simulink model "openWaterModel"  (R2020a)
settings: Solver=FixedStepAuto  StartTime=0.0  StopTime=inf  FixedStep=Ts  RelTol=1e-3  EnableMultiTasking=on
values from neighbouring files (symbols this model uses):
  ctrlMap =     [init_Kite.mat]
  Ts = 0.01    [init_Kite.mat]
undefined symbols (not defined in the file or in its folder): initializeBussesFromBlock, IO397, standard
libraries: xpcutilitieslib x172, hdlsllib x100, simulink x36, dspsigops x13, slrtlib x4, xpcseriallib x3, speedgoatlib_fpga_analog_io x2, xpcrtudplib x2, speedgoatlib_fpga_dio x1, speedgoatlib_fpga_quadrature x1, speedgoatlib_IO581 x1, speedgoatlib_fpga x1
(part 1 of 4)
settings Model: SimulationMode=external  Creator=MAE-VermillionLab  LastModifiedBy=mae-vermillionlab
settings SolverCC: ConcurrentTasks=on  AutoInsertRateTranBlk=on
settings DataIOCC: SaveFormat=StructureWithTime
settings OptimizationCC: BlockReduction=off  OptimizeBlockIOStorage=off
settings HardwareCC: ProdBitPerPointer=32  ProdBitPerSizeT=32  ProdBitPerPtrDiffT=32  ProdLargestAtomicFloat=None  ProdWordSize=32  ProdLongLongMode=on  ProdHWDeviceType=Generic->32-bit x86 compatible
settings RTWCC: Description=Simulink Real-Time  SystemTargetFile=slrt.tlc  TLCOptions=-axPCMaxOverloads=30 -axPCOverLoadLen=2 -axPCStartupFlag=5  TemplateMakefile=slrt_default_tmf  CodeExecutionProfiling=on  RTWCompilerOptimization=on
settings SimulinkRealTimeCC: SupportVariableSizeSignals=on  RL32LogBufSizeModifier=1e8  xPCConcurrentTasks=on

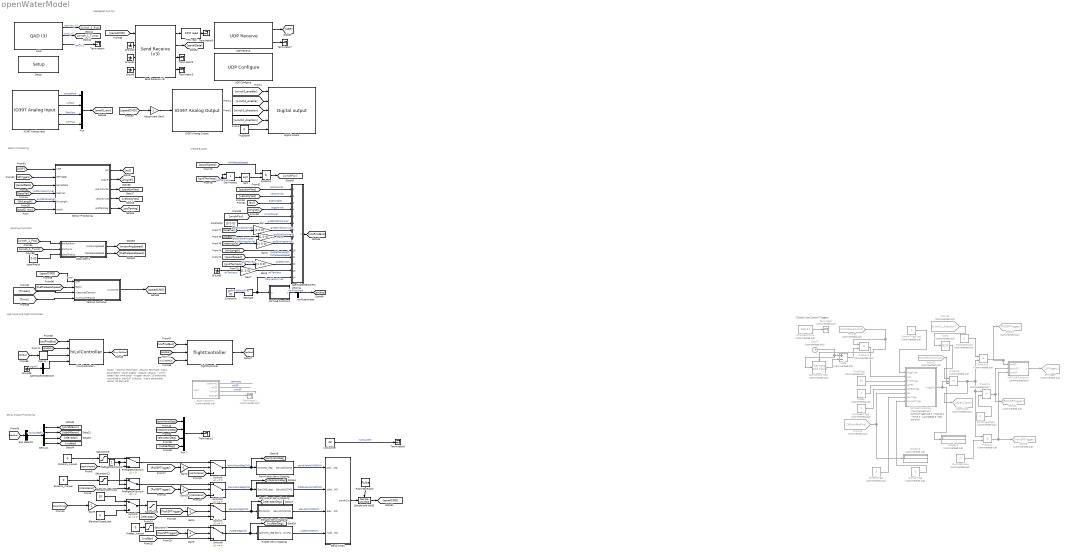
== system openWaterModel ==
  note: Spooling Controller
  note: Speedgoat Comms
  note: Create Busses
  note: High Level and Flight Controllers
  note: ControlTriggType
      | 0 - Manual
      | 1 - Time
      | 2 - LAS Speed
      | 3 - Enc position
  note: Closed Loop Control Triggers
  note: Serial Output Processing
  note: Sensor Processing
  note: Inputs:
      | - position estimate
      | - velocity estimate
      | - basis parameters
      | - euler angles
      | - angular velocity
      | - winch speed (last time step)
      | - trigger vector (10 constants controlled by the GUI)
      |
      |
      | Outputs:
      | -  basis parameter vector (10 element)
  Add3 : Sum  Commented=on  Inputs=+-
  Adjustment Gain1 : Gain
  Bus Selector : BusSelector  OutputSignals=ctrlSurfDefl
  Clock7 : Clock  Commented=on
  Constant3 : Constant  Value=[0 0 0]'
  Constant4 : Constant  Value=[0 0 0]'
  ControlTriggType : Constant  Commented=on  Value=0
  Demux1 : Demux
  Digital output : speedgoatlib_fpga_dio/Digital output  id=1  chan=[1:5]  init=[0]  reset=[0]  vectorizeInput=off  ts=Ts  pciSlot=-1  board=IO397-50k
      settings: SourceProductName=Simulink Real-Time: Speedgoat I/O Driver Library
  Display2 : Display  Commented=on
  Display3 : Display  Commented=on
  Dot Product : DotProduct  InputSameDT=on  OutDataTypeStr=Inherit: Inherit via internal rule
  Elevator Servo Mapping : Subsystem
  ElevatorClosedLoop : Constant  Value=0
  ElevatorOpenLoop : Constant  Value=10
  EncPosTrigg : Constant  Commented=on  Value=3
  "Euler setpoints " : Subsystem  Commented=on  mask{EulerSP=[0 0 0]}
      mask prompts: EulerSP "Euler Setpoints"
  "FIFO read " : xpcseriallib/FIFO read   maxsize=1024  minsize=1  usedelimiter=off  delimiter=13  outputtype=8 bit uint null terminated  enable=off  enableout=off  sampletime=Ts
      settings: SourceProductBaseCode=XP
  From22 : From  Commented=on  GotoTag=WinchPowerActual
  From23 : From  Commented=on  GotoTag=WinchAbsPos
  From31 : From  Commented=on  GotoTag=winch1_direction
  From33 : From  Commented=on  GotoTag=WinchPowerActual
  Gain{,1..2,6..7} (5 alike) : Gain  Gain=[1 0 0]'
  Gain{3..5,9,20} (5 alike) : Gain  Gain=-1
  Goto23 : Goto  Commented=on  GotoTag=RollSPTrigger
  Goto24 : Goto  Commented=on  GotoTag=PitchSPTrigger
  Goto25 : Goto  Commented=on  GotoTag=YawSPTrigger
  Ground{,1..2,5..6} (5 alike) : Ground
  IO397 Analog Input : speedgoatlib_fpga_analog_io/IO397 Analog Input  id=1  chan=[1:4]  range=+-5 V  trigger=Initiator  ts=Ts  pciSlot=-1  board=IO397-50k
      settings: SourceProductName=Simulink Real-Time: Speedgoat I/O Blockset
  IO397 Analog Output : speedgoatlib_fpga_analog_io/IO397 Analog Output  id=1  chan=[1]  initVal=0  resetVal=0  ts=Ts  pciSlot=-1  board=IO397-50k  span=+5 V
      settings: SourceProductName=Simulink Real-Time: Speedgoat I/O Driver Library
  LASspeedTrigg : Constant  Commented=on
  MATLAB Function1 : MATLAB Function  Commented=on  TreatAsAtomicUnit=on
  MATLAB Function2 : MATLAB Function  TreatAsAtomicUnit=on
  MATLAB Function4 : MATLAB Function  Commented=on  TreatAsAtomicUnit=on
  ManualTrigg : Constant  Commented=on  Value=0
  Memory : Memory
  Mux : Mux
  Mux7 : Mux
  NOT2 : Logic  Commented=on  Operator=NOT  IconShape=distinctive  AllPortsSameDT=off  OutDataTypeStr=boolean
  OpenClose : Goto  Commented=on  GotoTag=OpenClose
  PAileron_manual : Constant  Value=0  OutDataTypeStr=int8
  PitchOpenClose : Constant  Commented=on  Value=0
  Port Aileron Servo Mapping : Subsystem
  PreflightRollControl : Constant
  PreflightRollSwitch : Switch  Criteria=u2 > Threshold
  PreflightSAilSwitch : Switch  Criteria=u2 > Threshold
  Product{1..4} (4 alike) : Product  Commented=on
  Product5 : Product  Commented=on  Inputs=3
  Product6 : Product
  Pulse Generator : DiscretePulseGenerator  PulseType=Time based  Period=0.04  PulseWidth=50
  QAD : speedgoatlib_fpga_quadrature/QAD (3)  id=1  board=IO397-50k  chan=[2]  resetOnStart=on  ts=Ts  pciSlot=-1  operatingMode=Quadrature decoder  indexControlMode=Ignore index  resolution=1x  stepsPerRevolution=[1200]  latchMode=Disabled  interpolatePosition=off  invertAB=off  showClearPositionInput=off  showClearIndexFoundInput=off  showPositionOutput=on  showTurnOutput=on  showSpeedOutput=on  showDirectionOutput=off  showIndexFoundOutput=off
      settings: SourceProductName=Simulink Real-Time: Speedgoat I/O Driver Library
  Reshape : Reshape  OutputDimensionality=Column vector (2-D)
  RollOpenClose : Constant  Commented=on  Value=0
  Rudder Servo Mapping : Subsystem
  Rudder_manual : Constant  Value=0  OutDataTypeStr=int8
  SAileron_manual : Constant  Value=0  OutDataTypeStr=int8
  SPTrigger : Goto  Commented=on  GotoTag=SPTriggers
  Sample and Hold : dspsigops/Sample and Hold  Commented=on  trig=Rising edge  initCond=0  latchinput=off
  Sample and Hold3 : dspsigops/Sample and Hold  trig=Rising edge  initCond=0  latchinput=off
  Saturation{5..7,13} (4 alike) : Saturate  UpperLimit=30  LowerLimit=-30
  "Send Receive (v3) " : speedgoatlib_IO581/Send Receive (v3)   parModuleId=1  parSlot=-1  parModuleType=IO581  parTransceiver12=RS485 Half-Duplex  parTransceiver34=RS232  parTransceiver1=RS485 Half-Duplex  parAutoTurnaround1=off  parTurnaroundDelay1=0  parStandardBaud1=on  parBaudrate1=115200  parBaudDivisor1=1  parSamplingRate1=16x (standard)  parPrescale1=off  parCalcBaud1=7812500  parParity1=None  parDataBits1=8  parStopBits1=1  parTxTrigLvl1=1  parRxTrigLvl1=1  parHandshake1=none  parRtsHysteresis1=0  parXon1=17  parXoff1=19  parTxSwFifoSize1=1024  parTxSwFifoType1=8 bit uint null terminated  parRxSwFifoSize1=1024  parTransceiver2=RS485 Half-Duplex  parAutoTurnaround2=off  parTurnaroundDelay2=0  parStandardBaud2=on  parBaudrate2=115200  parBaudDivisor2=1  parSamplingRate2=16x (standard)  parPrescale2=off  parCalcBaud2=7812500  parParity2=None  parDataBits2=8  parStopBits2=1  parTxTrigLvl2=1  parRxTrigLvl2=1  parHandshake2=none  parRtsHysteresis2=0  parXon2=17  parXoff2=19  parTxSwFifoSize2=1024  parTxSwFifoType2=8 bit uint null terminated  parRxSwFifoSize2=1024  parTransceiver3=RS232  parAutoTurnaround3=off  parTurnaroundDelay3=0  parStandardBaud3=on  parBaudrate3=115200  parBaudDivisor3=1  parSamplingRate3=16x (standard)  parPrescale3=off  parCalcBaud3=7812500  parParity3=None  parDataBits3=8  parStopBits3=1  parTxTrigLvl3=1  parRxTrigLvl3=8  parHandshake3=none  parRtsHysteresis3=0  parXon3=17  parXoff3=19  parTxSwFifoSize3=1024  parTxSwFifoType3=8 bit uint null terminated  parRxSwFifoSize3=1024  parTransceiver4=RS232  parAutoTurnaround4=off  parTurnaroundDelay4=0  parStandardBaud4=on  parBaudrate4=115200  parBaudDivisor4=1  parSamplingRate4=16x (standard)  parPrescale4=off  parCalcBaud4=7812500  parParity4=None  parDataBits4=8  parStopBits4=1  parTxTrigLvl4=1  parRxTrigLvl4=1  parHandshake4=none  parRtsHysteresis4=0  parXon4=17  parXoff4=19  parTxSwFifoSize4=1024  parTxSwFifoType4=8 bit uint null terminated  parRxSwFifoSize4=1024
      settings: SourceProductName=Simulink Real-Time: Speedgoat Library
  Sensor Processing : Subsystem
  Serial CMD1 : Subsystem
  Setup : speedgoatlib_fpga/Setup/Setup  board=IO397-50k  id=1  device_id=1  frontIO=None  rearIO=None  bitstreamFile=init_Kite.mat  rev=1.0  timestamp_string=21/04/20 11:41:53  fpgaFreq=75 MHz  fpgaTick=13.33 ns  ProgSpiFlash=off  ProgBPIFlash=off  pciSlot=-1  PullRPort0=pull-up 3.3V  VioPort0=3.3V  PullRPort1=pull-up 3.3V  VioPort1=3.3V  PullRPort2=pull-up 3.3V  VioPort2=3.3V  PullRPort3=pull-up 3.3V  VioPort3=3.3V  PullRPort4=pull-up 3.3V  VioPort4=3.3V  PullRPort5=pull-up 3.3V  VioPort5=3.3V  PullRPort6=pull-up 3.3V  VioPort6=3.3V  PullRPort15=pull-up 3.3V  PullRPort31=pull-up 3.3V  PullRPort47=pull-up 3.3V  PullRPort63=pull-up 3.3V
      settings: SourceProductName=Simulink Real-Time: Speedgoat Library
  Sqrt : Sqrt  SaturateOnIntegerOverflow=on
  Star Aileron Servo Mapping : Subsystem
  Subsystem1 : Subsystem
  Switch{6..9,15} (5 alike) : Switch
  Terminator : Terminator  Commented=on
  Terminator1 : Terminator  Commented=on
  Terminator{2..8} (7 alike) : Terminator
  TimeTrigg : Constant  Commented=on  Value=10
  TrigDigital : Constant  Value=0
  UDP Configure : xpcrtudplib/UDP Configure  Priority=-1  IpAddress=30.30.30.1  SubnetMask=255.255.255.0  Gateway=0.0.0.0  PciBus=15  PciSlot=0  PciFunction=0  ID=1  tune=0  disable=off  enableMulticast=off  MulticastIpAddress={}  MulticastMask={}
      settings: SourceProductBaseCode=XP
  UDP Receive : xpcrtudplib/UDP Receive  ipAddressVal=30.30.30.1  localPort=25001  rcvWidth=14  rcvFmAny=off  fmAddress=30.30.30.2  rcvMulticast=off  multicastAddress={}  maxUDPQueue=8  sampleTime=Ts
  WinchStartTime : Constant  Commented=on  Value=316.61
  YawOpenClose : Constant  Commented=on  Value=0
  envOpenWater : BusCreator  InitFcn=initializeBussesFromBlock(gcb)  Inputs=1
  flightController : flightController_cl/flightController  SystemSampleTime=-1  Latency=0  AutoFrameSizeCalculation=off
      settings: PropagateVariantConditions=on
  hiLvlController1 : hiLvlController_cl/hiLvlController  SystemSampleTime=-1  Latency=0  AutoFrameSizeCalculation=off
  openWaterGndStnCtrl : BusCreator  InitFcn=initializeBussesFromBlock(gcb)  Inputs=1
  openWaterSensorProcessing : Subsystem  InitFcn=initializeBussesFromBlock(gcb);
  runCounter : Constant  Value=22
  speed : Constant  Commented=on
  spoolRadius : Constant  Value=0.05
  tension controller : Subsystem
  wires:
  QAD/1 -> [winch_1_Pos]  "position_w1"
  QAD/2 -> [winch_1_Turns]  "turns_w1"
  QAD/3 -> Terminator4/1  "rpm_w1"
  "Send Receive (v3) "/2 -> [serialData]
  "Send Receive (v3) "/1 -> "FIFO read "/1
  Ground2/1 -> "Send Receive (v3) "/2
  Ground1/1 -> "Send Receive (v3) "/3
  "FIFO read "/1 -> Terminator6/1
  Ground/1 -> "Send Receive (v3) "/4
  "Send Receive (v3) "/4 -> Terminator3/1
  "Send Receive (v3) "/3 -> Terminator5/1
  UDP Receive/2 -> Terminator7/1
  UDP Receive/1 -> [UDP]
  [portAileron] -> Switch6/3
  [rudder] -> Switch8/3
  [elevator] -> Switch7/3
  Switch8/1 -> [rudderDeg], Rudder Servo Mapping/1(YawCMD_deg)  "rudderDegCMD"
  Switch6/1 -> [portAileronDeg], Port Aileron Servo Mapping/1(RollCMD_deg)  "portAileronDegCMD"
  [RollSPTrigger] -> Gain3/1
  Rudder_manual/1 -> Saturation7/1
  Switch7/1 -> [elevatorDeg], Elevator Servo Mapping/1(PitchCMD)  "elevatorDegCMD"
  Saturation7/1 -> Switch8/1
  [PitchSPTrigger] -> Gain4/1
  [YawSPTrigger] -> Gain5/1
  Saturation5/1 -> Switch7/1
  runCounter/1 -> Terminator8/1  "runCounter"
  Switch9/1 -> Saturation5/1
  EncPosTrigg/1 -> MATLAB Function4/7(posTrigg)
  ControlTriggType/1 -> MATLAB Function4/1(triggType)
  From23/1 -> Display3/1, MATLAB Function4/6(pos)
  speed/1 -> MATLAB Function4/4(speed)
  LASspeedTrigg/1 -> MATLAB Function4/5(speedTrigg)
  TimeTrigg/1 -> MATLAB Function4/3(timeTrigg)
  Clock7/1 -> Sample and Hold/1, Add3/1
  Add3/1 -> Product1/2
  Product1/1 -> MATLAB Function4/2(clck)
  YawOpenClose/1 -> Product4/2
  PitchOpenClose/1 -> Product3/2
  RollOpenClose/1 -> Product2/1
  Product4/1 -> Goto25/1, MATLAB Function1/3(yawSP)
  Product3/1 -> MATLAB Function1/2(pitchSP), Goto24/1
  Product2/1 -> MATLAB Function1/1(rollSP), Goto23/1
  MATLAB Function1/1(y) -> SPTrigger/1
  ManualTrigg/1 -> MATLAB Function4/8(manualTrigg)
  From31/1 -> NOT2/1
  NOT2/1 -> Product5/1
  MATLAB Function4/1(triggON) -> Display2/1, Product5/2
  Product5/1 -> OpenClose/1, Product4/1, Product3/1, Product2/2
  Gain3/1 -> Switch6/2
  Gain4/1 -> Switch7/2
  Gain5/1 -> Switch8/2
  From33/1 -> Sample and Hold/Trigger, Product1/1
  From22/1 -> Product5/3
  WinchStartTime/1 -> Terminator/1
  Sample and Hold/1 -> Add3/2
  [OpenClose] -> Gain9/1
  ElevatorOpenLoop/1 -> Switch9/1
  ElevatorClosedLoop/1 -> Switch9/3
  Gain9/1 -> Switch9/2
  Port Aileron Servo Mapping/1(ServoRollCMD) -> Serial CMD1/1("portAileronCMD ")  "portAileronCMDPWM"
  Elevator Servo Mapping/1(ServoPitchCMD) -> Serial CMD1/3(elevatorCMD)  "elevatorCMDPWM"
  Rudder Servo Mapping/1(ServoYawCMD) -> Serial CMD1/4(rudderCMD)  "rudderCMDPWM"
  [portAileron] -> PreflightRollSwitch/3
  Saturation6/1 -> PreflightRollSwitch/1
  PAileron_manual/1 -> Saturation6/1
  PreflightRollSwitch/1 -> Switch6/1
  Serial CMD1/1(serialOut) -> Sample and Hold3/1
  Sample and Hold3/1 -> [serialCMD]
  Constant4/1 -> Reshape/1  "flowVelocityVec"
  [snsProcBus] -> hiLvlController1/1
  [snsProcBus] -> flightController/1
  hiLvlController1/1 -> [hiLvlCtrlBus]
  [hiLvlCtrlBus] -> flightController/3
  flightController/1 -> [ctrlBus]
  [ctrlBus] -> Memory/1
  Memory/1 -> hiLvlController1/3
  Ground6/1 -> openWaterGndStnCtrl/1  "signal1"
  Reshape/1 -> openWaterSensorProcessing/14(flowVelocityVec), MATLAB Function2/1(u)  "flowVelocityVec"
  MATLAB Function2/1(y) -> envOpenWater/1  "vhclFlowVecs"
  [envBus] -> hiLvlController1/2
  [envBus] -> flightController/2
  [gndTenVecs] -> Dot Product/1, Dot Product/2  "gndTenVecs"
  Dot Product/1 -> Sqrt/1
  Sqrt/1 -> Product6/2
  [spoolSpeed] -> Product6/1  "thrReleaseSpeeds"
  Product6/1 -> [wnchPwr]
  [serialCMD] -> "Send Receive (v3) "/1
  Adjustment Gain1/1 -> IO397 Analog Output/1
  TrigDigital/1 -> Digital output/5
  [winch2_direction] -> Digital output/4
  [winch2_enable] -> Digital output/2
  [speedCMD] -> Adjustment Gain1/1
  [winch1_enable] -> Digital output/1
  [winch1_direction] -> Digital output/3
  "Euler setpoints "/2(rollSP) -> ?  "rollSP"
  "Euler setpoints "/3(YawSP) -> ?  "yawSP"
  "Euler setpoints "/1(setPoints) -> ?  "setPoints"
  "Euler setpoints "/4(PitchSP) -> Terminator1/1
  [UDP] -> Sensor Processing/1(UDP)
  [SPTriggers] -> Sensor Processing/2(SPTrigger)
  [serialData] -> Sensor Processing/3(SerialData)
  Sensor Processing/1(eul) -> [eul]
  Sensor Processing/2(angVel) -> [angVel]
  Sensor Processing/3(positionVec) -> [positionVec]
  Sensor Processing/4(velocityVec) -> [velocityVec]
  Sensor Processing/5(gndTenMag) -> [gndTenMag]
  [boatVel] -> Sensor Processing/4(boatVel)  "gndStnVelocityVec"
  [thrLength] -> Sensor Processing/5(thrLength)  "avgTetherLength"
  Pulse Generator/1 -> Sample and Hold3/Trigger
  [ctrlBus] -> Bus Selector/1
  Bus Selector/1 -> Demux1/1  "<ctrlSurfDefl>"
  Demux1/1 -> [portAileron]
  Demux1/2 -> [stbdAileron]
  Demux1/3 -> [elevator]
  Demux1/4 -> [rudder]
  [winch_1_Pos] -> Subsystem1/1(encPosRaw)
  [winch_1_Turns] -> Subsystem1/2(encTurns)
  spoolRadius/1 -> Subsystem1/3(spoolRadius)
  Subsystem1/1(motorAngSpeed) -> [motorAngSpeed]
  Subsystem1/2(theReleaseSpeed) -> [theReleaseSpeed]
  IO397 Analog Input/2 -> Mux/2  "LCRaw"
  IO397 Analog Input/1 -> Mux/1  "torqueRaw"
  IO397 Analog Input/3 -> Mux/3  "flowRaw"
  IO397 Analog Input/4 -> Mux/4  "currRaw"
  Mux/1 -> [anaIO_raw]
  [anaIO_raw] -> Sensor Processing/6(anaIO)
  [starAileron] -> PreflightSAilSwitch/3
  Gain20/1 -> Switch15/2
  PreflightSAilSwitch/1 -> Switch15/1
  SAileron_manual/1 -> Saturation13/1
  Saturation13/1 -> PreflightSAilSwitch/1
  Switch15/1 -> [stbdAileronDeg], Star Aileron Servo Mapping/1(StarCMD_deg)  "starAileronDegCMD"
  Star Aileron Servo Mapping/1(ServoRollCMD) -> Serial CMD1/2(stbdAileronCMD)  "stbdAileronCMDPWM"
  [RollSPTrigger] -> Gain20/1
  PreflightRollControl/1 -> PreflightSAilSwitch/2, PreflightRollSwitch/2
  [starAileron] -> Switch15/3
  [stbdAileronDeg] -> Mux7/2
  [portAileronDeg] -> Mux7/1
  [elevatorDeg] -> Mux7/3
  [rudderDeg] -> Mux7/4
  Mux7/1 -> Terminator2/1
  [spoolCMD] -> tension controller/1(uref)  "uref"
  [theReleaseSpeed] -> tension controller/2(fbCtrl)
  tension controller/1(wnchCMD) -> [speedCMD]
  [Tmeas] -> tension controller/3(measuredTension)
  [Tmin] -> tension controller/4(minimumTension)
  [positionVec] -> openWaterSensorProcessing/1(positionVec)  "positionVec"
  [velocityVec] -> openWaterSensorProcessing/2(velocityVec)  "velocityVec"
  [eul] -> openWaterSensorProcessing/3(eulerAngles)  "eulerAngles"
  [angVel] -> openWaterSensorProcessing/4(angularVel)  "angularVel"
  [wnchPwr] -> openWaterSensorProcessing/5(winchPower)  "winchPower"
  Constant3/1 -> openWaterSensorProcessing/6(gndStnPositionVec)  "gndStnPositionVec"
  [boatVel] -> Gain/1  "gndStnVelocityVec"
  [boatEul] -> Gain1/1  "gndStnEulerAngles"
  [boatAngVel] -> Gain2/1  "gndStnAngularVel"
  [thrLength] -> openWaterSensorProcessing/10(avgTetherLength)  "avgTetherLength"
  [spoolSpeed] -> openWaterSensorProcessing/11(thrReleaseSpeeds)  "thrReleaseSpeeds"
  [gndTenVecs] -> Gain6/1  "gndTenVecs"
  Ground5/1 -> Gain7/1  "airTenVecs"
  openWaterSensorProcessing/1(Out1) -> [snsProcBus]
  envOpenWater/1 -> [envBus]
  openWaterGndStnCtrl/1 -> hiLvlController1/4
  Gain/1 -> openWaterSensorProcessing/7(gndStnVelocityVec)  "gndStnVelocityVec"
  Gain1/1 -> openWaterSensorProcessing/8(gndStnEulerAngles)  "gndStnEulerAngles"
  Gain2/1 -> openWaterSensorProcessing/9(gndStnAngularVel)  "gndStnAngularVel"
  Gain6/1 -> openWaterSensorProcessing/12(gndTenVecs)  "gndTenVecs"
  Gain7/1 -> openWaterSensorProcessing/13(airTenVecs)  "airTenVecs"

== system openWaterModel/Elevator Servo Mapping ==
  note: Negative gain added due to servo orientation
  PitchCMD : Inport
  1-D Lookup Table : Lookup_n-D  NumberOfTableDimensions=1  BreakpointsForDimension1=ctrlMap.El(2,82:182)  Table=ctrlMap.El(1,82:182)  InternalRulePriority=Speed  RndMeth=Simplest  InputSameDT=on
  Add : Sum
  Add1 : Sum
  Bias 1 : Constant  Value=7.2
  Bias 2 : Constant  Value=0.2802
  Display : Display
  Display1 : Display
  Gain : Gain  Gain=1.138
  Gain4 : Gain  Gain=-1
  ServoPitchCMD : Outport
  wires:
  Gain4/1 -> 1-D Lookup Table/1
  Add/1 -> Gain/1
  PitchCMD/1 -> Display1/1, Gain4/1
  1-D Lookup Table/1 -> Add/1
  Bias 1/1 -> Add/2  "PitchServoBias"
  Gain/1 -> Add1/1
  Add1/1 -> Display/1, ServoPitchCMD/1
  Bias 2/1 -> Add1/2  "PitchServoBias_extra"

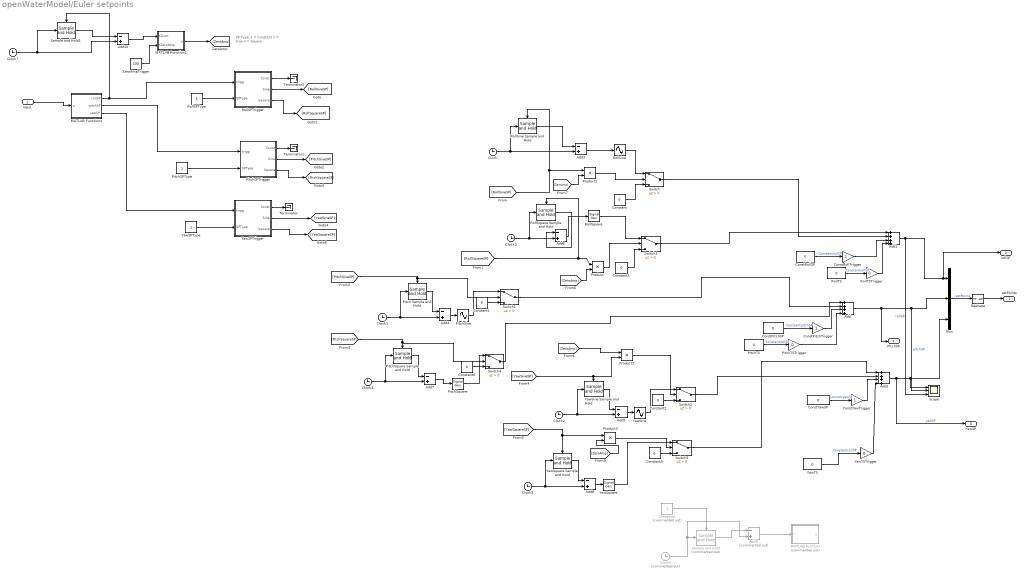
== system openWaterModel/Euler setpoints  ==
  note: SP Type:
      | 1 = Constant
      | 2 = Sine
      | 3 = Square
  Input : Inport
  Add : Sum  Inputs=++++
  Add1 : Sum  Inputs=++++
  Add{3..8,10} (7 alike) : Sum  Inputs=-+
  Add2 : Sum  Inputs=++++
  Add9 : Sum  Commented=on  Inputs=-+
  Clock{,1..5,7} (7 alike) : Clock
  Clock6 : Clock  Commented=on
  ConstPitchSP : Constant  Value=0
  ConstPitchTrigger : Gain
  ConstRollSP : Constant  Value=0
  ConstRollTrigger : Gain
  ConstYawSP : Constant  Value=0
  ConstYawTrigger : Gain
  Constant{,1..5} (6 alike) : Constant  Value=0
  Constant6 : Constant  Commented=on
  MATLAB Function : MATLAB Function  Commented=on  TreatAsAtomicUnit=on
  MATLAB Function1 : MATLAB Function  TreatAsAtomicUnit=on
  MATLAB Function4 : MATLAB Function  TreatAsAtomicUnit=on
  Mux : Mux  Inputs=3
  Pitch Sample and Hold : dspsigops/Sample and Hold  trig=Rising edge  initCond=0  latchinput=off
  PitchSPTrigger : MATLAB Function  TreatAsAtomicUnit=on
  PitchSPType : Constant
  PitchSine : Sin  TimeSource=Use external signal  Amplitude=40  Frequency=2.0944  Phase=5
  PitchSquare : SignalGenerator  WaveForm=square  TimeSource=Use external signal  Frequency=3.1416  Units=rad/sec
  PitchSquare Sample and Hold : dspsigops/Sample and Hold  trig=Rising edge  initCond=0  latchinput=off
  PitchTS : Constant  Value=0
  PitchTSTrigger : Gain  Gain=0
  Product{,1..3} (4 alike) : Product
  Reshape : Reshape  OutputDimensionality=Column vector (2-D)
  RollSPTrigger : MATLAB Function  TreatAsAtomicUnit=on
  RollSPType : Constant
  RollSine : Sin  TimeSource=Use external signal  Amplitude=30  Frequency=0.83776
  RollSine Sample and Hold : dspsigops/Sample and Hold  trig=Rising edge  initCond=0  latchinput=off
  RollSquare : SignalGenerator  WaveForm=square  TimeSource=Use external signal  Amplitude=0  Frequency=6.2832  Units=rad/sec
  RollSquare Sample and Hold : dspsigops/Sample and Hold  trig=Rising edge  initCond=0  latchinput=off
  RollTS : Constant  Value=0
  RollTSTrigger : Gain  Gain=0
  Sample and Hold : dspsigops/Sample and Hold  Commented=on  trig=Rising edge  initCond=0  latchinput=off
  Sample and Hold1 : dspsigops/Sample and Hold  trig=Rising edge  initCond=0  latchinput=off
  Scope : Scope  NumInputPorts=3
  Switch{,1..5} (6 alike) : Switch  Criteria=u2 > Threshold
  Terminator : Terminator
  Terminator1 : Terminator
  Terminator2 : Terminator
  YawSPTrigger : MATLAB Function  TreatAsAtomicUnit=on
  YawSPType : Constant
  YawSine : Sin  TimeSource=Use external signal  Amplitude=60  Frequency=0.83776  Phase=-0.877
  YawSine Sample and Hold : dspsigops/Sample and Hold  trig=Rising edge  initCond=0  latchinput=off
  YawSquare : SignalGenerator  WaveForm=square  TimeSource=Use external signal  Frequency=3.1416  Units=rad/sec
  YawSquare Sample and Hold : dspsigops/Sample and Hold  trig=Rising edge  initCond=0  latchinput=off
  YawTS : Constant  Value=0
  YawTSTrigger : Gain  Gain=0
  ZeroAmpTrigger : Constant  Value=100
  setPoints : Outport
  rollSP : Outport  Port=2
  YawSP : Outport  Port=3
  PitchSP : Outport  Port=4
  wires:
  Mux/1 -> Reshape/1  "setPoints"
  Reshape/1 -> setPoints/1
  Switch1/1 -> Add/2
  Switch4/1 -> Add/1
  ConstPitchSP/1 -> ConstPitchTrigger/1  "ConstantpitchSP"
  Switch3/1 -> Add1/1
  ConstRollSP/1 -> ConstRollTrigger/1  "ConstantrollSP"
  Switch2/1 -> Add2/2
  Switch5/1 -> Add2/1
  ConstYawSP/1 -> ConstYawTrigger/1  "ConstntyawSP"
  Add2/1 -> YawSP/1, Mux/3, Scope/1  "yawSP"
  Add/1 -> PitchSP/1, Mux/2, Scope/2  "pitchSP"
  Add1/1 -> Scope/3, Mux/1, rollSP/1  "rollSP"
  RollTSTrigger/1 -> Add1/4
  PitchTSTrigger/1 -> Add/4
  RollTS/1 -> RollTSTrigger/1  "ConstantrollSP"
  PitchTS/1 -> PitchTSTrigger/1  "ConstantrollSP"
  Switch/1 -> Add1/2
  Add3/1 -> RollSine/1
  Constant/1 -> Switch/3
  RollSine Sample and Hold/1 -> Add3/1
  RollSine/1 -> Switch/1
  Clock/1 -> Add3/2, RollSine Sample and Hold/1
  Pitch Sample and Hold/1 -> Add4/1
  Add4/1 -> PitchSine/1
  Constant1/1 -> Switch1/3
  [PitchSineSP] -> Switch1/2, Pitch Sample and Hold/Trigger
  PitchSine/1 -> Switch1/1
  Clock1/1 -> Add4/2, Pitch Sample and Hold/1
  [YawSineSP] -> Product2/2, YawSine Sample and Hold/Trigger
  Constant2/1 -> Switch2/3
  YawSine/1 -> Switch2/1
  YawSine Sample and Hold/1 -> Add5/1
  Add5/1 -> YawSine/1
  Clock2/1 -> Add5/2, YawSine Sample and Hold/1
  Clock3/1 -> Add6/2, RollSquare Sample and Hold/1
  RollSquare Sample and Hold/1 -> Add6/1
  Add6/1 -> RollSquare/1
  [RollSquareSP] -> Product/1, RollSquare Sample and Hold/Trigger
  Constant3/1 -> Switch3/3
  RollSquare/1 -> Switch3/1
  [PitchSquareSP] -> Switch4/2, PitchSquare Sample and Hold/Trigger
  Constant4/1 -> Switch4/3
  PitchSquare/1 -> Switch4/1
  PitchSquare Sample and Hold/1 -> Add7/1
  Add7/1 -> PitchSquare/1
  Clock4/1 -> Add7/2, PitchSquare Sample and Hold/1
  Clock5/1 -> Add8/2, YawSquare Sample and Hold/1
  YawSquare Sample and Hold/1 -> Add8/1
  [YawSquareSP] -> Product3/1, YawSquare Sample and Hold/Trigger
  Add8/1 -> YawSquare/1
  YawSquare/1 -> Switch5/1
  Constant5/1 -> Switch5/3
  Constant6/1 -> Sample and Hold/Trigger
  Sample and Hold/1 -> Add9/1
  Clock6/1 -> Sample and Hold/1, Add9/2
  Add9/1 -> MATLAB Function/1(t)
  YawTS/1 -> YawTSTrigger/1  "ConstantrollSP"
  YawTSTrigger/1 -> Add2/4
  ConstRollTrigger/1 -> Add1/3
  ConstPitchTrigger/1 -> Add/3
  ConstYawTrigger/1 -> Add2/3
  [RollSineSP] -> Product1/1, RollSine Sample and Hold/Trigger
  Input/1 -> MATLAB Function4/1(u)
  RollSPType/1 -> RollSPTrigger/2(SPType)
  MATLAB Function4/1(rollSP) -> RollSPTrigger/1(trigg), Sample and Hold1/Trigger
  PitchSPType/1 -> PitchSPTrigger/2(SPType)
  MATLAB Function4/2(pitchSP) -> PitchSPTrigger/1(trigg)
  YawSPType/1 -> YawSPTrigger/2(SPType)
  MATLAB Function4/3(yawSP) -> YawSPTrigger/1(trigg)
  RollSPTrigger/2(Sine) -> [RollSineSP]
  RollSPTrigger/3(Square) -> [RollSquareSP]
  YawSPTrigger/3(Square) -> [YawSquareSP]
  YawSPTrigger/2(Sine) -> [YawSineSP]
  PitchSPTrigger/3(Square) -> [PitchSquareSP]
  PitchSPTrigger/2(Sine) -> [PitchSineSP]
  Clock7/1 -> Sample and Hold1/1, Add10/2
  Sample and Hold1/1 -> Add10/1
  Add10/1 -> MATLAB Function1/1(tZcurr)
  ZeroAmpTrigger/1 -> MATLAB Function1/2(tZeroAmp)
  MATLAB Function1/1(y) -> [ZeroAmp]
  Product/1 -> Switch3/2
  [ZeroAmp] -> Product/2
  Product1/1 -> Switch/2
  [ZeroAmp] -> Product1/2
  YawSPTrigger/1(Const) -> Terminator/1
  PitchSPTrigger/1(Const) -> Terminator1/1
  [ZeroAmp] -> Product2/1
  [ZeroAmp] -> Product3/2
  Product3/1 -> Switch5/2
  Product2/1 -> Switch2/2
  RollSPTrigger/1(Const) -> Terminator2/1

== system openWaterModel/Port Aileron Servo Mapping ==
  RollCMD_deg : Inport
  Add2 : Sum
  Bias : Constant  Value=0
  ServoRollCMD : Outport
  wires:
  Bias/1 -> Add2/2  "RollServoBias"
  RollCMD_deg/1 -> Add2/1
  Add2/1 -> ServoRollCMD/1

== system openWaterModel/Rudder Servo Mapping ==
  YawCMD_deg : Inport
  1-D Lookup Table : Lookup_n-D  NumberOfTableDimensions=1  BreakpointsForDimension1=ctrlMap.vStab(2,60:170)  Table=ctrlMap.vStab(1,60:170)  InternalRulePriority=Speed  RndMeth=Simplest  InputSameDT=on
  Add : Sum
  Bias 1 : Constant  Value=0
  ServoYawCMD : Outport
  wires:
  YawCMD_deg/1 -> 1-D Lookup Table/1
  Bias 1/1 -> Add/2  "PitchServoBias"
  1-D Lookup Table/1 -> Add/1
  Add/1 -> ServoYawCMD/1

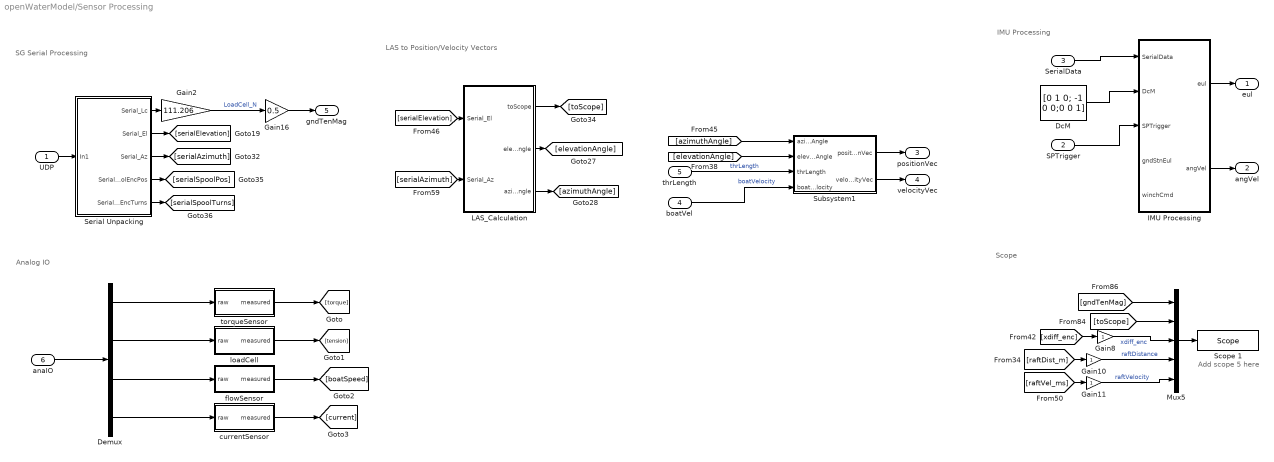
== system openWaterModel/Sensor Processing ==
  note: Analog IO
  note: LAS to Position/Velocity Vectors
  note: IMU Processing
  note: Scope
  note: SG Serial Processing
  note: Add scope 5 here
  UDP : Inport
  SPTrigger : Inport  Port=2
  SerialData : Inport  Port=3
  boatVel : Inport  Port=4
  thrLength : Inport  Port=5
  anaIO : Inport  Port=6
  DcM : Constant  Value=[0 1 0; -1 0 0;0 0 1]
  Demux : Demux
  Gain10 : Gain
  Gain11 : Gain
  Gain16 : Gain  Gain=0.5
  Gain2 : Gain  Gain=111.206
  Gain8 : Gain
  IMU Processing : Subsystem
  LAS_Calculation : Subsystem
  Mux5 : Mux  Inputs=5
  Scope 1 : slrtlib/Displays and Logging/Scope   scopeno=5  scopetype=Target  autostart=on  viewmode=Numerical  formatstr='%15.6f'  grid=on  ylimits=[0,0]  nosamples=scopeSamples  noprepostsamples=0  interleave=scopeDecimaton  triggermode=FreeRun  triggersignal=1  trigsignalfromport=off  triggerlevel=0.0  triggerslope=Either  triggerscope=1  triggersample=0  filename=data.dat  mode=Lazy  writesize=512  autorestart=off  dynamicfilemode=off  maxwritefilesize=512*1024^2
  Serial Unpacking : Subsystem
  Subsystem1 : Subsystem
  currentSensor : Subsystem
  flowSensor : Subsystem
  loadCell : Subsystem
  torqueSensor : Subsystem
  eul : Outport
  angVel : Outport  Port=2
  positionVec : Outport  Port=3
  velocityVec : Outport  Port=4
  gndTenMag : Outport  Port=5
  wires:
  [raftDist_m] -> Gain10/1
  Gain8/1 -> Mux5/3  "xdiff_enc"
  DcM/1 -> IMU Processing/2(DcM)
  Serial Unpacking/4(Serial_SpoolEncPos) -> [serialSpoolPos]
  [serialElevation] -> LAS_Calculation/1(Serial_El)
  Serial Unpacking/1(Serial_Lc) -> Gain2/1
  [toScope] -> Mux5/2
  Serial Unpacking/3(Serial_Az) -> [serialAzimuth]
  [elevationAngle] -> Subsystem1/2(elevationAngle)
  [serialAzimuth] -> LAS_Calculation/2(Serial_Az)
  Mux5/1 -> Scope 1/1
  [xdiff_enc] -> Gain8/1
  LAS_Calculation/3(azimuthAngle) -> [azimuthAngle]
  UDP/1 -> Serial Unpacking/1(In1)
  IMU Processing/2(angVel) -> angVel/1
  Gain2/1 -> Gain16/1  "LoadCell_N"
  [gndTenMag] -> Mux5/1
  Gain10/1 -> Mux5/4  "raftDistance"
  Subsystem1/2(velocityVec) -> velocityVec/1
  LAS_Calculation/2(elevationAngle) -> [elevationAngle]
  Gain16/1 -> gndTenMag/1
  [raftVel_ms] -> Gain11/1
  Gain11/1 -> Mux5/5  "raftVelocity"
  LAS_Calculation/1(toScope) -> [toScope]
  boatVel/1 -> Subsystem1/4(boatVelocity)  "boatVelocity"
  SPTrigger/1 -> IMU Processing/3(SPTrigger)
  thrLength/1 -> Subsystem1/3(thrLength)  "thrLength"
  [azimuthAngle] -> Subsystem1/1(azimuthAngle)
  Serial Unpacking/5(Serial_SpoolEncTurns) -> [serialSpoolTurns]
  Serial Unpacking/2(Serial_El) -> [serialElevation]
  IMU Processing/1(eul) -> eul/1
  SerialData/1 -> IMU Processing/1(SerialData)
  Subsystem1/1(positionVec) -> positionVec/1
  anaIO/1 -> Demux/1
  Demux/1 -> torqueSensor/1(raw)
  torqueSensor/1(measured) -> [torque]
  loadCell/1(measured) -> [tension]
  flowSensor/1(measured) -> [boatSpeed]
  currentSensor/1(measured) -> [current]
  Demux/4 -> currentSensor/1(raw)
  Demux/3 -> flowSensor/1(raw)
  Demux/2 -> loadCell/1(raw)

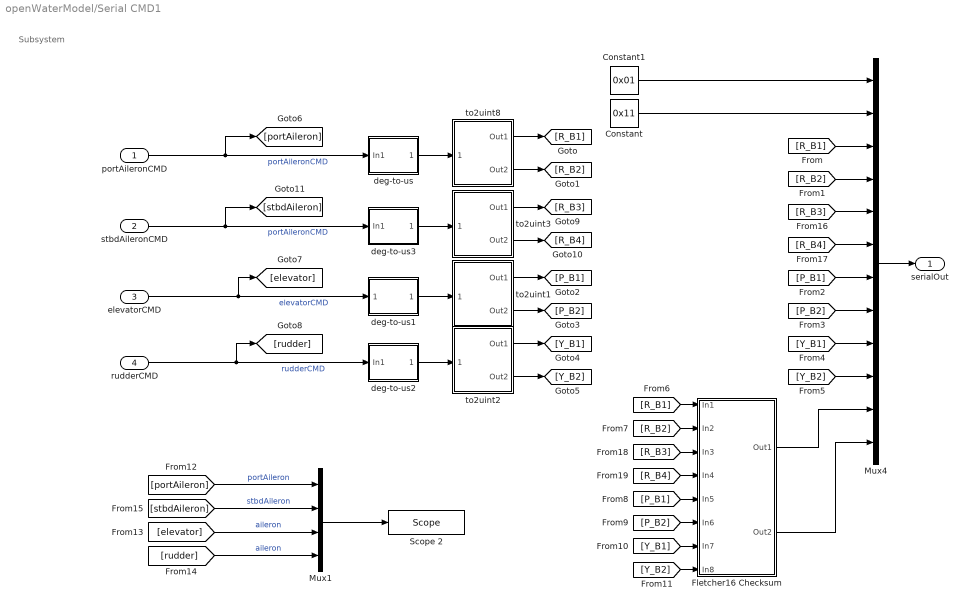
== system openWaterModel/Serial CMD1 ==
  note: Subsystem
  "portAileronCMD " : Inport
  stbdAileronCMD : Inport  Port=2
  elevatorCMD : Inport  Port=3
  rudderCMD : Inport  Port=4
  Constant : Constant  Value=0x11  OutDataTypeStr=uint8
  Constant1 : Constant  Value=0x01  OutDataTypeStr=uint8
  Fletcher16 Checksum : Subsystem
  Mux1 : Mux
  Mux4 : Mux  Inputs=12
  Scope 2 : slrtlib/Displays and Logging/Scope   scopeno=2  scopetype=Target  autostart=on  viewmode=Graphical sliding  formatstr='%15.6f'  grid=on  ylimits=[-60,60]  nosamples=scopeSamples  noprepostsamples=0  interleave=scopeDecimaton  triggermode=FreeRun  triggersignal=1  trigsignalfromport=off  triggerlevel=0.0  triggerslope=Either  triggerscope=1  triggersample=0  filename=data.dat  mode=Lazy  writesize=512  autorestart=off  dynamicfilemode=off  maxwritefilesize=512*1024^2
  deg-to-us : Subsystem
  deg-to-us1 : Subsystem
  deg-to-us2 : Subsystem
  deg-to-us3 : Subsystem
  to2uint1 : Subsystem
  to2uint2 : Subsystem
  to2uint3 : Subsystem
  to2uint8 : Subsystem
  serialOut : Outport
  wires:
  elevatorCMD/1 -> [elevator], deg-to-us1/1(pitchCMD)  "elevatorCMD"
  Constant/1 -> Mux4/2
  rudderCMD/1 -> [rudder], deg-to-us2/1(In1)  "rudderCMD"
  "portAileronCMD "/1 -> [portAileron], deg-to-us/1(In1)  "portAileronCMD"
  Constant1/1 -> Mux4/1
  deg-to-us1/1(" ") -> to2uint1/1(" ")
  to2uint8/1(Out1) -> [R_B1]
  to2uint8/2(Out2) -> [R_B2]
  to2uint1/1(Out1) -> [P_B1]
  to2uint1/2(Out2) -> [P_B2]
  to2uint2/1(Out1) -> [Y_B1]
  to2uint2/2(Out2) -> [Y_B2]
  [R_B1] -> Mux4/3
  [R_B2] -> Mux4/4
  [R_B1] -> Fletcher16 Checksum/1(In1)
  [R_B2] -> Fletcher16 Checksum/2(In2)
  Mux4/1 -> serialOut/1
  deg-to-us2/1(" ") -> to2uint2/1(" ")
  deg-to-us/1(" ") -> to2uint8/1(" ")
  [portAileron] -> Mux1/1  "portAileron"
  [elevator] -> Mux1/3  "aileron"
  [rudder] -> Mux1/4  "aileron"
  [stbdAileron] -> Mux1/2  "stbdAileron"
  to2uint3/2(Out2) -> [R_B4]
  stbdAileronCMD/1 -> [stbdAileron], deg-to-us3/1(In1)  "portAileronCMD"
  deg-to-us3/1(" ") -> to2uint3/1(" ")
  to2uint3/1(Out1) -> [R_B3]
  [P_B1] -> Mux4/7
  [P_B2] -> Mux4/8
  [Y_B1] -> Mux4/9
  [Y_B2] -> Mux4/10
  [R_B4] -> Mux4/6
  [R_B3] -> Mux4/5
  [P_B1] -> Fletcher16 Checksum/5(In5)
  [P_B2] -> Fletcher16 Checksum/6(In6)
  [Y_B1] -> Fletcher16 Checksum/7(In7)
  [Y_B2] -> Fletcher16 Checksum/8(In8)
  [R_B3] -> Fletcher16 Checksum/3(In3)
  [R_B4] -> Fletcher16 Checksum/4(In4)
  Fletcher16 Checksum/1(Out1) -> Mux4/11
  Fletcher16 Checksum/2(Out2) -> Mux4/12
  Mux1/1 -> Scope 2/1

== system openWaterModel/Star Aileron Servo Mapping ==
  StarCMD_deg : Inport
  Add2 : Sum
  Bias : Constant  Value=0
  ServoRollCMD : Outport
  wires:
  Bias/1 -> Add2/2  "RollServoBias"
  StarCMD_deg/1 -> Add2/1
  Add2/1 -> ServoRollCMD/1

== system openWaterModel/Subsystem1 ==
  encPosRaw : Inport
  encTurns : Inport  Port=2
  spoolRadius : Inport  Port=3
  Difference : simulink/Discrete/Difference  ICPrevInput=0.0  OutMin=[]  OutMax=[]  OutDataType=fixdt(1, 16)  OutScaling=2^-10  DoSatur=off
  Difference1 : simulink/Discrete/Difference  ICPrevInput=0.0  OutMin=[]  OutMax=[]  OutDataType=fixdt(1, 16)  OutScaling=2^-10  DoSatur=off
  Direction : Gain
  Direction1 : Gain
  EncPosEstimation : Subsystem
  Gain2 : Gain  Gain=1/Ts
  Gain6 : Gain  Gain=1/Ts
  Low Pass Filter : TransferFcn  Denominator=[0.02 1]
  Low Pass Filter1 : TransferFcn  Denominator=[0.02 1]
  motorAngSpeed : Outport
  theReleaseSpeed : Outport  Port=2
  wires:
  EncPosEstimation/2(ThrLength) -> [thrLength]  "theLength"
  Direction/1 -> theReleaseSpeed/1
  Gain6/1 -> Direction1/1
  [thrLength] -> Difference/1
  Gain2/1 -> Direction/1
  EncPosEstimation/1(angPos_rad) -> [motorAng_rad]
  Difference1/1 -> Low Pass Filter1/1
  Low Pass Filter1/1 -> Gain6/1
  Difference/1 -> Low Pass Filter/1
  [motorAng_rad] -> Difference1/1
  Low Pass Filter/1 -> Gain2/1
  encTurns/1 -> EncPosEstimation/2(encTurns)
  Direction1/1 -> motorAngSpeed/1
  encPosRaw/1 -> EncPosEstimation/1(encPosRaw)
  spoolRadius/1 -> EncPosEstimation/3(spoolRadius)

== system openWaterModel/openWaterSensorProcessing ==
  positionVec : Inport
  velocityVec : Inport  Port=2
  eulerAngles : Inport  Port=3
  angularVel : Inport  Port=4
  winchPower : Inport  Port=5
  gndStnPositionVec : Inport  Port=6
  gndStnVelocityVec : Inport  Port=7
  gndStnEulerAngles : Inport  Port=8
  gndStnAngularVel : Inport  Port=9
  avgTetherLength : Inport  Port=10
  thrReleaseSpeeds : Inport  Port=11
  gndTenVecs : Inport  Port=12
  airTenVecs : Inport  Port=13
  flowVelocityVec : Inport  Port=14
  Bus Creator : BusCreator  Inputs=14
  Out1 : Outport
  wires:
  flowVelocityVec/1 -> Bus Creator/14
  gndStnEulerAngles/1 -> Bus Creator/8
  gndTenVecs/1 -> Bus Creator/12
  gndStnAngularVel/1 -> Bus Creator/9
  positionVec/1 -> Bus Creator/1
  gndStnVelocityVec/1 -> Bus Creator/7
  thrReleaseSpeeds/1 -> Bus Creator/11
  gndStnPositionVec/1 -> Bus Creator/6
  avgTetherLength/1 -> Bus Creator/10
  airTenVecs/1 -> Bus Creator/13
  velocityVec/1 -> Bus Creator/2
  winchPower/1 -> Bus Creator/5
  angularVel/1 -> Bus Creator/4
  Bus Creator/1 -> Out1/1
  eulerAngles/1 -> Bus Creator/3

== system openWaterModel/tension controller ==
  note: FF
  note: FB
  uref : Inport
  fbCtrl : Inport  Port=2
  measuredTension : Inport  Port=3
  minimumTension : Inport  Port=4
  Add2 : Sum
  Add8 : Sum  Inputs=+-
  Add9 : Sum  Inputs=+-
  FilteredPIDController1 : Subsystem  mask{Kp=1, Kd=0, tau=1, Ki=0}
      mask prompts: Kp "Proportional Gain"; Kd "Derivative Gain"; tau "Time constant"; Ki "Integral Gain"
  FilteredPIDController2 : Subsystem  mask{Kp=1, Kd=0, tau=1, Ki=0}
      mask prompts: Kp "Proportional Gain"; Kd "Derivative Gain"; tau "Time constant"; Ki "Integral Gain"
  Min : MinMax  Inputs=2
  wnchCMD : Outport
  wires:
  Add8/1 -> FilteredPIDController1/1(del_u)
  FilteredPIDController1/1(y) -> Add2/2
  uref/1 -> Add8/1, Add2/1
  Add9/1 -> FilteredPIDController2/1(del_u)  "e"
  measuredTension/1 -> Add9/1
  Add2/1 -> Min/1
  Min/1 -> wnchCMD/1
  FilteredPIDController2/1(y) -> Min/2  "spl"
  minimumTension/1 -> Add9/2
  fbCtrl/1 -> Add8/2

== system openWaterModel/Sensor Processing/IMU Processing ==
  SerialData : Inport
  DcM : Inport  Port=2
  SPTrigger : Inport  Port=3
  gndStnEul : Inport  Port=4
  winchCmd : Inport  Port=5
  Controller1 : Subsystem  Commented=on  mask{ctrlSurfDefMax=45, pitchKP=1, yawKP=1, rollKP=1}
      mask prompts: ctrlSurfDefMax "Max Ctrlsurf def"; pitchKP "pitch Kp"; yawKP "yaw Kp"; rollKP "roll Kp"
  "Kite Measurements " : Subsystem
  Reshape : Reshape  OutputDimensionality=Column vector (2-D)
  Terminator : Terminator
  Terminator1 : Terminator
  Terminator2 : Terminator
  eul : Outport
  angVel : Outport  Port=2
  wires:
  SerialData/1 -> "Kite Measurements "/1(serialData)
  DcM/1 -> "Kite Measurements "/2(DcM)
  SPTrigger/1 -> Terminator/1
  "Kite Measurements "/3(angVel) -> angVel/1
  "Kite Measurements "/2(eul) -> Reshape/1
  Reshape/1 -> eul/1
  gndStnEul/1 -> "Kite Measurements "/3(gndStnEul)
  winchCmd/1 -> "Kite Measurements "/4(winchCmd)
  "Kite Measurements "/1(kiteMeasure) -> Terminator1/1  "KiteYaw"
  "Kite Measurements "/4(MC_rawData) -> Terminator2/1

== system openWaterModel/Sensor Processing/LAS_Calculation ==
  Serial_El : Inport
  Serial_Az : Inport  Port=2
  Add2 : Sum
  Add3 : Sum
  Az_deg_calib : Constant  Value=-348.5775
  Constant : Constant  Value=360
  Constant2 : Constant  Value=360
  El_deg_calib : Constant  Value=-246.6236
  Gain : Gain  Gain=360/8192
  Gain1 : Gain  Gain=360/8192
  Gain2 : Gain  Gain=pi/180
  Gain3 : Gain  Gain=pi/180
  Gain4 : Gain  Gain=180/pi
  Gain5 : Gain  Gain=180/pi
  LAS Measurement Corrections : MATLAB Function  TreatAsAtomicUnit=on
  Mod : Math  Operator=mod  SaturateOnIntegerOverflow=on
  Mod1 : Math  Operator=mod  SaturateOnIntegerOverflow=on
  Mux : Mux
  ifOutsideBounds : MATLAB Function  TreatAsAtomicUnit=on
  ifOutsideBounds1 : MATLAB Function  TreatAsAtomicUnit=on
  toScope : Outport
  elevationAngle : Outport  Port=2
  azimuthAngle : Outport  Port=3
  wires:
  Gain/1 -> Mod/1
  Constant2/1 -> Mod1/2
  Constant/1 -> Mod/2
  Mod/1 -> Add2/1
  Serial_Az/1 -> Gain1/1
  Mod1/1 -> Add3/1
  Gain1/1 -> Mod1/1
  ifOutsideBounds/1(y) -> [elEncoder]  "El_deg"
  Add3/1 -> ifOutsideBounds1/1(u)  "Az_deg"
  Serial_El/1 -> Gain/1
  Gain2/1 -> LAS Measurement Corrections/1(elev_encoder)
  Gain3/1 -> LAS Measurement Corrections/2(azi_encoder)
  LAS Measurement Corrections/2(azi) -> Gain5/1
  LAS Measurement Corrections/1(elev) -> Gain4/1
  Gain4/1 -> [elevation], elevationAngle/1  "elevationAngle"
  Gain5/1 -> [azimuth], azimuthAngle/1  "azimuthAngle"
  Mux/1 -> toScope/1
  Az_deg_calib/1 -> Add3/2
  El_deg_calib/1 -> Add2/2
  Add2/1 -> ifOutsideBounds/1(u)  "El_deg"
  ifOutsideBounds1/1(y) -> [azEncoder]  "Az_deg"
  [elEncoder] -> Gain2/1
  [azEncoder] -> Gain3/1
  [elEncoder] -> Mux/3
  [azEncoder] -> Mux/4
  [elevation] -> Mux/1
  [azimuth] -> Mux/2

== system openWaterModel/Sensor Processing/Serial Unpacking ==
  In1 : Inport
  Demux : Demux  Outputs=14
  Display{1..9} (9 alike) : Display
  Subsystem : Subsystem
  Subsystem1 : Subsystem
  binary2double1 : Subsystem
  binary2double2 : Subsystem
  binary2double5 : Subsystem
  Serial_Lc : Outport
  Serial_El : Outport  Port=2
  Serial_Az : Outport  Port=3
  Serial_SpoolEncPos : Outport  Port=4
  Serial_SpoolEncTurns : Outport  Port=5
  wires:
  Demux/6 -> Subsystem/2(In2)
  Demux/5 -> Subsystem/1(In1)
  In1/1 -> Demux/1
  Subsystem/1(Double) -> Display7/1, Serial_El/1
  Demux/8 -> Subsystem1/2(In2)
  Demux/7 -> Subsystem1/1(In1)
  Subsystem1/1(Double) -> Display8/1, Serial_Az/1
  Demux/1 -> binary2double5/1(In1)
  Demux/2 -> binary2double5/2(In2)
  Demux/3 -> binary2double5/3(In3)
  Demux/4 -> binary2double5/4(In4)
  binary2double5/1(Double) -> Display2/1, Serial_Lc/1  "Yaw Rate"
  Demux/9 -> binary2double1/1(In3), Display1/1
  Demux/10 -> binary2double1/2(In4), Display3/1
  Demux/11 -> binary2double2/1(In1), Display4/1
  Demux/12 -> binary2double2/2(In2), Display5/1
  binary2double1/1(Double) -> Serial_SpoolEncPos/1
  Demux/13 -> binary2double2/3(In3), Display6/1
  Demux/14 -> binary2double2/4(In4), Display9/1
  binary2double2/1(Double) -> Serial_SpoolEncTurns/1

== system openWaterModel/Sensor Processing/Subsystem1 ==
  azimuthAngle : Inport
  elevationAngle : Inport  Port=2
  thrLength : Inport  Port=3
  boatVelocity : Inport  Port=4
  Reshape : Reshape  OutputDimensionality=Column vector (2-D)
  Reshape1 : Reshape  OutputDimensionality=Column vector (2-D)
  Subsystem1 : Subsystem
  positionVec : Outport
  velocityVec : Outport  Port=2
  wires:
  Subsystem1/1(positionVec) -> Reshape/1
  Reshape/1 -> positionVec/1
  Reshape1/1 -> velocityVec/1
  Subsystem1/2(velocityVec) -> Reshape1/1
  azimuthAngle/1 -> Subsystem1/2(azLAS)
  elevationAngle/1 -> Subsystem1/1(elLAS)
  thrLength/1 -> Subsystem1/3(thrLength)
  boatVelocity/1 -> Subsystem1/4(boatVelocity)

== system openWaterModel/Sensor Processing/currentSensor ==
  raw : Inport
  Add : Sum
  Constant : Constant
  Gain : Gain
  measured : Outport
  wires:
  Gain/1 -> Add/1
  Constant/1 -> Add/2
  Add/1 -> measured/1
  raw/1 -> Gain/1

== system openWaterModel/Sensor Processing/flowSensor ==
  raw : Inport
  Add : Sum
  Constant : Constant
  Gain : Gain
  measured : Outport
  wires:
  Gain/1 -> Add/1
  Constant/1 -> Add/2
  Add/1 -> measured/1
  raw/1 -> Gain/1

== system openWaterModel/Sensor Processing/loadCell ==
  raw : Inport
  Add : Sum
  Constant : Constant
  Gain : Gain
  measured : Outport
  wires:
  Gain/1 -> Add/1
  Constant/1 -> Add/2
  Add/1 -> measured/1
  raw/1 -> Gain/1

== system openWaterModel/Sensor Processing/torqueSensor ==
  raw : Inport
  Add : Sum
  Constant : Constant
  Gain : Gain
  measured : Outport
  wires:
  Gain/1 -> Add/1
  Constant/1 -> Add/2
  Add/1 -> measured/1
  raw/1 -> Gain/1

== system openWaterModel/Serial CMD1/Fletcher16 Checksum ==
  In1 : Inport
  In2 : Inport  Port=2
  In3 : Inport  Port=3
  In4 : Inport  Port=4
  In5 : Inport  Port=5
  In6 : Inport  Port=6
  In7 : Inport  Port=7
  In8 : Inport  Port=8
  Add : Sum  Inputs=++++++++
  Add1 : Sum  Inputs=++++++++
  Gain : Gain  Gain=6  OutDataTypeStr=uint8
  Gain1 : Gain  Gain=5  OutDataTypeStr=uint8
  Gain2 : Gain  Gain=4  OutDataTypeStr=uint8
  Gain3 : Gain  Gain=3  OutDataTypeStr=uint8
  Gain4 : Gain  Gain=2  OutDataTypeStr=uint8
  Gain5 : Gain  Gain=8  OutDataTypeStr=uint8
  Gain6 : Gain  Gain=7  OutDataTypeStr=uint8
  Out1 : Outport
  Out2 : Outport  Port=2
  wires:
  Add/1 -> Out1/1
  Add1/1 -> Out2/1
  Gain5/1 -> Add1/1
  Gain6/1 -> Add1/2
  Gain/1 -> Add1/3
  Gain1/1 -> Add1/4
  Gain2/1 -> Add1/5
  Gain3/1 -> Add1/6
  Gain4/1 -> Add1/7
  [B8] -> Add1/8
  [B7] -> Gain4/1
  [B6] -> Gain3/1
  [B5] -> Gain2/1
  [B4] -> Gain1/1
  [B3] -> Gain/1
  [B2] -> Gain6/1
  [B1] -> Gain5/1
  In8/1 -> [B8], Add/8
  In7/1 -> [B7], Add/7
  In6/1 -> [B6], Add/6
  In5/1 -> [B5], Add/5
  In4/1 -> [B4], Add/4
  In3/1 -> [B3], Add/3
  In2/1 -> [B2], Add/2
  In1/1 -> [B1], Add/1

== system openWaterModel/Serial CMD1/deg-to-us ==
  In1 : Inport
  Constant1 : Constant  Value=1500
  Gain : Gain  Gain=10
  Sum : Sum  Inputs=|++
  " " : Outport
  wires:
  Gain/1 -> Sum/1
  Constant1/1 -> Sum/2
  In1/1 -> Gain/1
  Sum/1 -> " "/1

== system openWaterModel/Serial CMD1/deg-to-us1 ==
  pitchCMD : Inport
  Constant1 : Constant  Value=1500
  Gain : Gain  Gain=10
  Sum : Sum  Inputs=|++
  " " : Outport
  wires:
  Sum/1 -> " "/1
  pitchCMD/1 -> Gain/1
  Constant1/1 -> Sum/2
  Gain/1 -> Sum/1

== system openWaterModel/Serial CMD1/deg-to-us2 ==
  In1 : Inport
  Constant1 : Constant  Value=1500
  Gain : Gain  Gain=10
  Sum : Sum  Inputs=|++
  " " : Outport
  wires:
  Gain/1 -> Sum/1
  Constant1/1 -> Sum/2
  In1/1 -> Gain/1
  Sum/1 -> " "/1

== system openWaterModel/Serial CMD1/deg-to-us3 ==
  In1 : Inport
  Constant1 : Constant  Value=1500
  Gain : Gain  Gain=10
  Sum : Sum  Inputs=|++
  " " : Outport
  wires:
  Gain/1 -> Sum/1
  Constant1/1 -> Sum/2
  In1/1 -> Gain/1
  Sum/1 -> " "/1

== system openWaterModel/Serial CMD1/to2uint1 ==
  " " : Inport
  Bit Packing 1 : xpcutilitieslib/Bit Packing   MaskBitPatterns={[0:7]}  MaskPackDataType=uint8  MaskPackDataSize=[1]
      settings: SourceProductBaseCode=XP
  Bit Packing 2 : xpcutilitieslib/Bit Packing   MaskBitPatterns={[0:7]}  MaskPackDataType=uint8  MaskPackDataSize=[1]
      settings: SourceProductBaseCode=XP
  Bit Shift2 : hdlsllib/Logic and Bit Operations/Bit Shift  mode=Shift Right Arithmetic  N=8
  Cast4 : DataTypeConversion  OutDataTypeStr=uint16
  Out1 : Outport
  Out2 : Outport  Port=2
  wires:
  Bit Packing 1/1 -> Out1/1
  " "/1 -> Cast4/1
  Cast4/1 -> Bit Packing 1/1, Bit Shift2/1
  Bit Packing 2/1 -> Out2/1
  Bit Shift2/1 -> Bit Packing 2/1

== system openWaterModel/Serial CMD1/to2uint2 ==
  " " : Inport
  Bit Packing 1 : xpcutilitieslib/Bit Packing   MaskBitPatterns={[0:7]}  MaskPackDataType=uint8  MaskPackDataSize=[1]
      settings: SourceProductBaseCode=XP
  Bit Packing 2 : xpcutilitieslib/Bit Packing   MaskBitPatterns={[0:7]}  MaskPackDataType=uint8  MaskPackDataSize=[1]
      settings: SourceProductBaseCode=XP
  Bit Shift2 : hdlsllib/Logic and Bit Operations/Bit Shift  mode=Shift Right Arithmetic  N=8
  Cast4 : DataTypeConversion  OutDataTypeStr=uint16
  Out1 : Outport
  Out2 : Outport  Port=2
  wires:
  Bit Shift2/1 -> Bit Packing 2/1
  Bit Packing 2/1 -> Out2/1
  Cast4/1 -> Bit Shift2/1, Bit Packing 1/1
  " "/1 -> Cast4/1
  Bit Packing 1/1 -> Out1/1

== system openWaterModel/Serial CMD1/to2uint3 ==
  " " : Inport
  Bit Packing 1 : xpcutilitieslib/Bit Packing   MaskBitPatterns={[0:7]}  MaskPackDataType=uint8  MaskPackDataSize=[1]
      settings: SourceProductBaseCode=XP
  Bit Packing 2 : xpcutilitieslib/Bit Packing   MaskBitPatterns={[0:7]}  MaskPackDataType=uint8  MaskPackDataSize=[1]
      settings: SourceProductBaseCode=XP
  Bit Shift2 : hdlsllib/Logic and Bit Operations/Bit Shift  mode=Shift Right Arithmetic  N=8
  Cast4 : DataTypeConversion  OutDataTypeStr=uint16
  Out1 : Outport
  Out2 : Outport  Port=2
  wires:
  Bit Shift2/1 -> Bit Packing 2/1
  Cast4/1 -> Bit Shift2/1, Bit Packing 1/1
  " "/1 -> Cast4/1
  Bit Packing 1/1 -> Out1/1
  Bit Packing 2/1 -> Out2/1

== system openWaterModel/Serial CMD1/to2uint8 ==
  " " : Inport
  Bit Packing 1 : xpcutilitieslib/Bit Packing   MaskBitPatterns={[0:7]}  MaskPackDataType=uint8  MaskPackDataSize=[1]
      settings: SourceProductBaseCode=XP
  Bit Packing 2 : xpcutilitieslib/Bit Packing   MaskBitPatterns={[0:7]}  MaskPackDataType=uint8  MaskPackDataSize=[1]
      settings: SourceProductBaseCode=XP
  Bit Shift2 : hdlsllib/Logic and Bit Operations/Bit Shift  mode=Shift Right Arithmetic  N=8
  Cast4 : DataTypeConversion  OutDataTypeStr=uint16
  Out1 : Outport
  Out2 : Outport  Port=2
  wires:
  Bit Shift2/1 -> Bit Packing 2/1
  Cast4/1 -> Bit Shift2/1, Bit Packing 1/1
  " "/1 -> Cast4/1
  Bit Packing 1/1 -> Out1/1
  Bit Packing 2/1 -> Out2/1

== system openWaterModel/Subsystem1/EncPosEstimation ==
  encPosRaw : Inport
  encTurns : Inport  Port=2
  spoolRadius : Inport  Port=3
  Add1 : Sum
  Cast To Double : DataTypeConversion  OutDataTypeStr=double
  Cast To Double1 : DataTypeConversion  OutDataTypeStr=double
  Gain : Gain  Gain=(2*pi)/1800
  Gain1 : Gain  Gain=1800
  Product : Product
  angPos_rad : Outport
  ThrLength : Outport  Port=2
  wires:
  Gain/1 -> angPos_rad/1, Product/1  "angPos_rad"
  Cast To Double/1 -> Add1/1
  Add1/1 -> Gain/1
  Gain1/1 -> Add1/2
  Product/1 -> ThrLength/1  "linearPos"
  encTurns/1 -> Cast To Double1/1
  spoolRadius/1 -> Product/2
  encPosRaw/1 -> Cast To Double/1
  Cast To Double1/1 -> Gain1/1

== system openWaterModel/tension controller/FilteredPIDController1 ==
  note: Anti-winding
  note: Tau with minimum
  del_u : Inport
  Abs : Abs
  Add1 : Sum  Inputs=+++
  Add2 : Sum  Inputs=+-
  Constant : Constant
  Constant1 : Constant  Value=0
  Constant2 : Constant
  Divide{1..4} (4 alike) : Product  Inputs=*/
  Int_reset : Constant  Value=0
  Integrator : Integrator
  Integrator3 : Integrator  ExternalReset=either
  Max : MinMax  Function=max  Inputs=2
  Product : Product
  Product1 : Product
  Switch : Switch  Threshold=30
  Weighted Sample Time : SampleTimeMath  TsampMathOp=Ts Only
  YawKd : Gain  Gain=0.05
  YawKi : Gain  Gain=0
  YawKp : Gain  Gain=0.3
  YawTau : Constant  Value=0.02
  const : Constant
  y : Outport
  wires:
  YawTau/1 -> Max/2
  Add1/1 -> [y], y/1
  const/1 -> Weighted Sample Time/1
  Weighted Sample Time/1 -> Max/1
  Max/1 -> [Tau]
  YawKd/1 -> Divide1/1
  Constant/1 -> YawKd/1
  [Tau] -> Divide1/2
  Divide1/1 -> Product/1
  Integrator/1 -> YawKp/1, Divide4/1, YawKi/1
  [Tau] -> Divide2/2
  Divide2/1 -> Integrator3/1
  Integrator3/1 -> Add1/2
  Product/1 -> Add1/1
  YawKp/1 -> Divide3/1
  Divide3/1 -> Add1/3
  [Tau] -> Divide3/2
  [Tau] -> Divide4/2
  del_u/1 -> Add2/1
  Divide4/1 -> Add2/2
  Add2/1 -> Product/2, Integrator/1
  [y] -> Abs/1
  Abs/1 -> Switch/2
  Constant1/1 -> Switch/1
  Constant2/1 -> Switch/3
  Switch/1 -> [stop_trig]
  YawKi/1 -> Product1/2
  [stop_trig] -> Product1/1
  Product1/1 -> Divide2/1
  Int_reset/1 -> Integrator3/2

== system openWaterModel/tension controller/FilteredPIDController2 ==
  note: Anti-winding
  note: Tau with minimum
  del_u : Inport
  Abs : Abs
  Add1 : Sum  Inputs=+++
  Add2 : Sum  Inputs=+-
  Constant : Constant
  Constant1 : Constant  Value=0
  Constant2 : Constant
  Divide{1..4} (4 alike) : Product  Inputs=*/
  Int_reset : Constant  Value=0
  Integrator : Integrator
  Integrator3 : Integrator  ExternalReset=either
  Max : MinMax  Function=max  Inputs=2
  PitchKd : Gain  Gain=0
  PitchKi : Gain  Gain=0
  PitchKp : Gain  Gain=2
  PitchTau : Constant  Value=0.05
  Product : Product
  Product1 : Product
  Switch : Switch  Threshold=30
  Weighted Sample Time : SampleTimeMath  TsampMathOp=Ts Only
  const : Constant
  y : Outport
  wires:
  PitchTau/1 -> Max/2
  Add1/1 -> [y], y/1
  const/1 -> Weighted Sample Time/1
  Weighted Sample Time/1 -> Max/1
  Max/1 -> [Tau]
  PitchKd/1 -> Divide1/1
  Constant/1 -> PitchKd/1
  [Tau] -> Divide1/2
  Divide1/1 -> Product/1
  Integrator/1 -> PitchKp/1, Divide4/1, PitchKi/1
  [Tau] -> Divide2/2
  Divide2/1 -> Integrator3/1
  Integrator3/1 -> Add1/2
  Product/1 -> Add1/1
  PitchKp/1 -> Divide3/1
  Divide3/1 -> Add1/3
  [Tau] -> Divide3/2
  [Tau] -> Divide4/2
  del_u/1 -> Add2/1
  Divide4/1 -> Add2/2
  Add2/1 -> Product/2, Integrator/1
  [y] -> Abs/1
  Abs/1 -> Switch/2
  Constant1/1 -> Switch/1
  Constant2/1 -> Switch/3
  Switch/1 -> [stop_trig]
  PitchKi/1 -> Product1/2
  [stop_trig] -> Product1/1
  Product1/1 -> Divide2/1
  Int_reset/1 -> Integrator3/2
